simulink model "Z_Systemidentifikation_PRBS"  (R2017b)
settings: Solver=ode45  StartTime=0.0  StopTime=1  MaxStep=5e-5  RelTol=1e-3  EnableMultiTasking=on
libraries: simulink x1
settings Model: Creator=jbaur  LastModifiedBy=jbaur
settings DataIOCC: ExternalInput=X1  SaveFormat=Array  SignalLoggingSaveFormat=ModelDataLogs  SignalLoggingName=sigsOut
settings OptimizationCC: ExpressionDepthLimit=2147483647  InitFltsAndDblsToZero=on  LifeSpan=inf
settings DebuggingCC: SaveWithParameterizedLinksMsg=none  SignalResolutionControl=TryResolveAllWithWarning  MultiTaskDSMMsg=warning  MultiTaskCondExecSysMsg=none  StateNameClashWarn=warning  SFUnexpectedBacktrackingDiag=warning  SFNoUnconditionalDefaultTransitionDiag=warning  SFExecutionAtInitializationDiag=none
settings HardwareCC: ProdBitPerPointer=32  ProdBitPerSizeT=32  ProdBitPerPtrDiffT=32  ProdLargestAtomicFloat=None  ProdIntDivRoundTo=Undefined  ProdEndianess=Unspecified  ProdWordSize=32  ProdHWDeviceType=32-bit Generic  TargetUnknown=on
settings ModelReferenceCC: PropagateSignalLabelsOutOfModel=off
settings CodeAppCC: StateflowObjectComments=on
settings GRTTargetCC: TargetFcnLib=ansi_tfl_tmw.mat  TargetLangStandard=C89/C90 (ANSI)  ModelReferenceCompliant=off  GeneratePreprocessorConditionals=Disable all  CombineOutputUpdateFcns=off  MatFileLogging=off  GRTInterface=on
settings ConfigComp: CovMetricSettings=dw  CovHtmlReporting=on  CovSaveCumulativeToWorkspaceVar=on  CovSaveSingleToWorkspaceVar=on  CovExternalEMLEnable=off  CovSFcnEnable=off

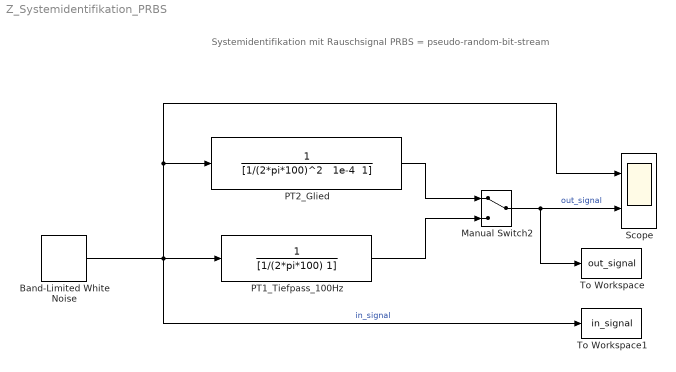
== system Z_Systemidentifikation_PRBS ==
  note: Systemidentifikation mit Rauschsignal
      | PRBS = pseudo-random-bit-stream
  Band-Limited White Noise : simulink/Sources/Band-Limited White Noise  Cov=[0.2]  Ts=1E-4  seed=[23341]
  Manual Switch2 : ManualSwitch
  PT1_Tiefpass_100Hz : TransferFcn  Denominator=[1/(2*pi*100) 1]
  PT2_Glied : TransferFcn  Denominator="[1/(2*pi*100)^2   1e-4  1]"
  Scope : Scope  NumInputPorts=2
  To Workspace : ToWorkspace  VariableName=out_signal  SaveFormat=Structure With Time  SampleTime=-1
  To Workspace1 : ToWorkspace  VariableName=in_signal  SaveFormat=Structure With Time  SampleTime=-1
  wires:
  PT2_Glied/1 -> Manual Switch2/1
  PT1_Tiefpass_100Hz/1 -> Manual Switch2/2
  Manual Switch2/1 -> Scope/2, To Workspace/1  "out_signal"
  Band-Limited White Noise/1 -> PT2_Glied/1, Scope/1, To Workspace1/1, PT1_Tiefpass_100Hz/1  "in_signal"
